simulink model "TST_ASMod_VolEff"  (R2016b)
settings: Solver=FixedStepDiscrete  StartTime=0.0  StopTime=simTime  FixedStep=sampleTime  RelTol=1e-3
values from neighbouring files (symbols this model uses):
  testCase = 1    [initTST_ASMod_VolEff_001.m]
libraries: simulink x5, UnitTest_Lib x3
settings Model: Creator=bianxuyin  LastModifiedBy=bianxuyin
settings DebuggingCC: SignalRangeChecking=error

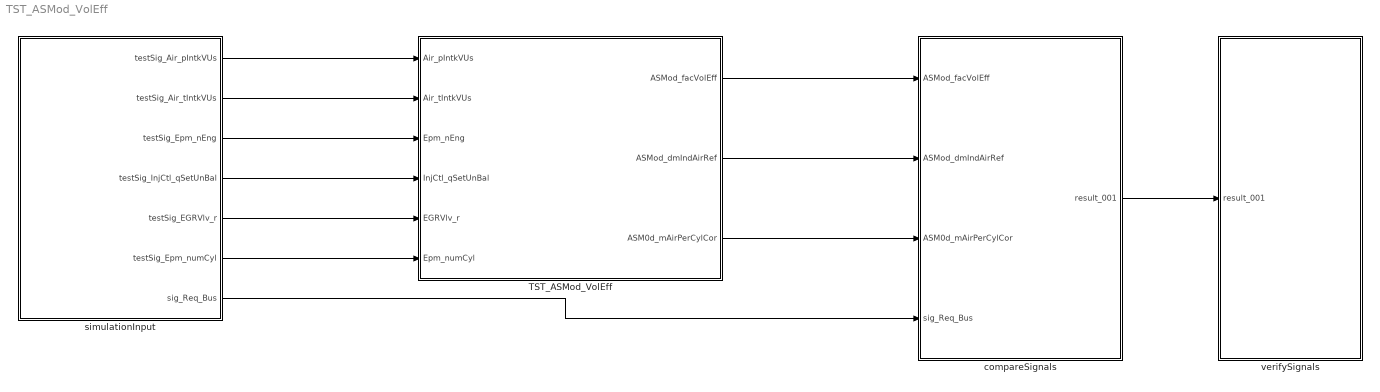
== system TST_ASMod_VolEff ==
  TST_ASMod_VolEff : Subsystem
  compareSignals : Subsystem
  simulationInput : Subsystem
  verifySignals : Subsystem
  wires:
  simulationInput/1(testSig_Air_pIntkVUs) -> TST_ASMod_VolEff/1(Air_pIntkVUs)
  simulationInput/2(testSig_Air_tIntkVUs) -> TST_ASMod_VolEff/2(Air_tIntkVUs)
  simulationInput/3(testSig_Epm_nEng) -> TST_ASMod_VolEff/3(Epm_nEng)
  simulationInput/4(testSig_InjCtl_qSetUnBal) -> TST_ASMod_VolEff/4(InjCtl_qSetUnBal)
  simulationInput/5(testSig_EGRVlv_r) -> TST_ASMod_VolEff/5(EGRVlv_r)
  simulationInput/6(testSig_Epm_numCyl) -> TST_ASMod_VolEff/6(Epm_numCyl)
  TST_ASMod_VolEff/1(ASMod_facVolEff) -> compareSignals/1(ASMod_facVolEff)
  TST_ASMod_VolEff/2(ASMod_dmIndAirRef) -> compareSignals/2(ASMod_dmIndAirRef)
  TST_ASMod_VolEff/3(ASM0d_mAirPerCylCor) -> compareSignals/3(ASM0d_mAirPerCylCor)
  simulationInput/7(sig_Req_Bus) -> compareSignals/4(sig_Req_Bus)
  compareSignals/1(result_001) -> verifySignals/1(result_001)

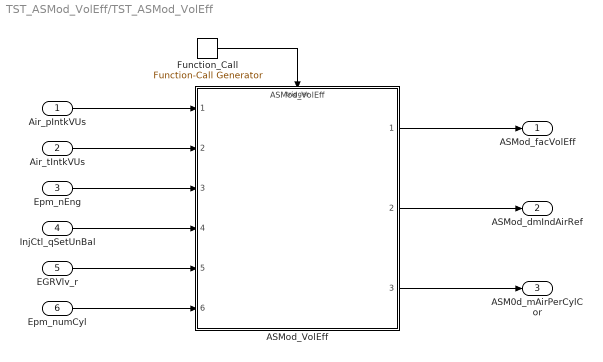
== system TST_ASMod_VolEff/TST_ASMod_VolEff ==
  Air_pIntkVUs : Inport
  Air_tIntkVUs : Inport  Port=2
  Epm_nEng : Inport  Port=3
  InjCtl_qSetUnBal : Inport  Port=4
  EGRVlv_r : Inport  Port=5
  Epm_numCyl : Inport  Port=6
  ASMod_VolEff : ModelReference  ModelNameDialog=ASMod_VolEff  SimulationMode=Normal  ModelReferenceVersion=1.20  TriggerPortName=function  TriggerPortTriggerType=function-call  TriggerPortStatesWhenEnabling=held
  Function_Call : simulink/Ports & Subsystems/Function-Call Generator  sample_time=sampleTime  numberOfIterations=1
  ASMod_facVolEff : Outport
  ASMod_dmIndAirRef : Outport  Port=2
  ASM0d_mAirPerCylCor : Outport  Port=3
  wires:
  Function_Call/1 -> ASMod_VolEff/Trigger
  Air_pIntkVUs/1 -> ASMod_VolEff/1
  Air_tIntkVUs/1 -> ASMod_VolEff/2
  Epm_nEng/1 -> ASMod_VolEff/3
  InjCtl_qSetUnBal/1 -> ASMod_VolEff/4
  EGRVlv_r/1 -> ASMod_VolEff/5
  Epm_numCyl/1 -> ASMod_VolEff/6
  ASMod_VolEff/1 -> ASMod_facVolEff/1
  ASMod_VolEff/2 -> ASMod_dmIndAirRef/1
  ASMod_VolEff/3 -> ASM0d_mAirPerCylCor/1

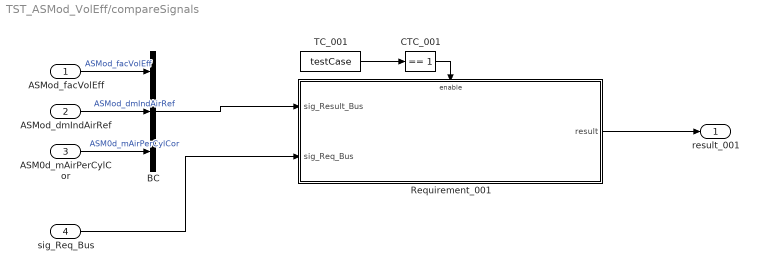
== system TST_ASMod_VolEff/compareSignals ==
  ASMod_facVolEff : Inport
  ASMod_dmIndAirRef : Inport  Port=2
  ASM0d_mAirPerCylCor : Inport  Port=3
  sig_Req_Bus : Inport  Port=4
  BC : BusCreator  Inputs=3
  CTC_001 : simulink/Logic and Bit Operations/Compare To Constant  relop===  const=1  OutDataTypeStr=boolean
  Requirement_001 : Subsystem
  TC_001 : Constant  Value=testCase
  result_001 : Outport
  wires:
  ASMod_facVolEff/1 -> BC/1  "ASMod_facVolEff"
  ASMod_dmIndAirRef/1 -> BC/2  "ASMod_dmIndAirRef"
  ASM0d_mAirPerCylCor/1 -> BC/3  "ASM0d_mAirPerCylCor"
  TC_001/1 -> CTC_001/1
  CTC_001/1 -> Requirement_001/Enable
  sig_Req_Bus/1 -> Requirement_001/2(sig_Req_Bus)
  BC/1 -> Requirement_001/1(sig_Result_Bus)
  Requirement_001/1(result) -> result_001/1

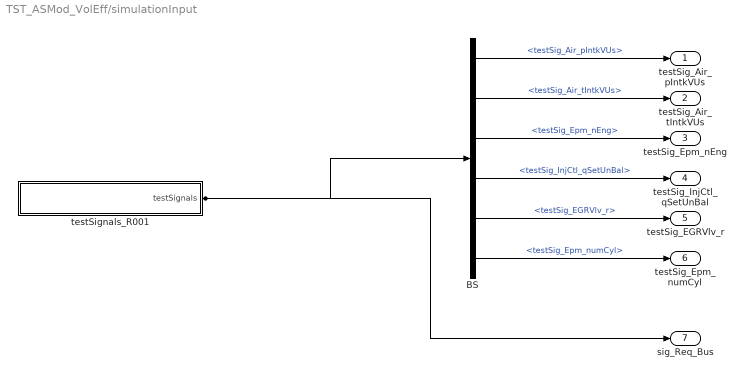
== system TST_ASMod_VolEff/simulationInput ==
  BS : BusSelector  OutputSignals=testSig_Air_pIntkVUs,testSig_Air_tIntkVUs,testSig_Epm_nEng,testSig_InjCtl_qSetUnBal,testSig_EGRVlv_r,testSig_Epm_numCyl
  testSignals_R001 : Subsystem
  testSig_Air_pIntkVUs : Outport
  testSig_Air_tIntkVUs : Outport  Port=2
  testSig_Epm_nEng : Outport  Port=3
  testSig_InjCtl_qSetUnBal : Outport  Port=4
  testSig_EGRVlv_r : Outport  Port=5
  testSig_Epm_numCyl : Outport  Port=6
  sig_Req_Bus : Outport  Port=7
  wires:
  BS/1 -> testSig_Air_pIntkVUs/1  "<testSig_Air_pIntkVUs>"
  BS/2 -> testSig_Air_tIntkVUs/1  "<testSig_Air_tIntkVUs>"
  BS/3 -> testSig_Epm_nEng/1  "<testSig_Epm_nEng>"
  BS/4 -> testSig_InjCtl_qSetUnBal/1  "<testSig_InjCtl_qSetUnBal>"
  BS/5 -> testSig_EGRVlv_r/1  "<testSig_EGRVlv_r>"
  BS/6 -> testSig_Epm_numCyl/1  "<testSig_Epm_numCyl>"
  testSignals_R001/1(testSignals) -> BS/1, sig_Req_Bus/1

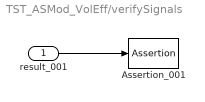
== system TST_ASMod_VolEff/verifySignals ==
  result_001 : Inport
  Assertion_001 : Assertion  Enabled=off
  wires:
  result_001/1 -> Assertion_001/1

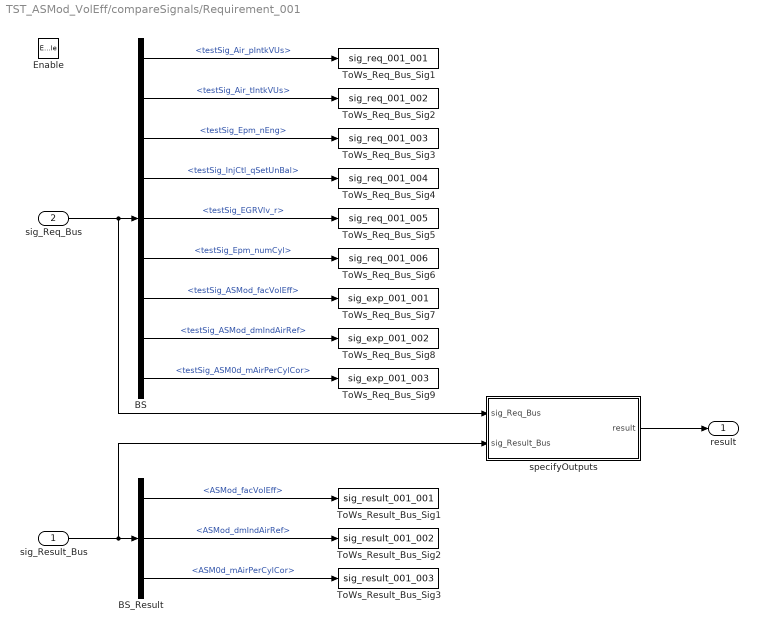
== system TST_ASMod_VolEff/compareSignals/Requirement_001 ==
  sig_Result_Bus : Inport
  sig_Req_Bus : Inport  Port=2
  Enable : EnablePort
  BS : BusSelector  OutputSignals=testSig_Air_pIntkVUs,testSig_Air_tIntkVUs,testSig_Epm_nEng,testSig_InjCtl_qSetUnBal,testSig_EGRVlv_r,testSig_Epm_numCyl,testSig_ASMod_facVolEff,testSig_ASMod_dmIndAirRef,testSig_ASM0d_mAirPerCylCor
  BS_Result : BusSelector  OutputSignals=ASMod_facVolEff,ASMod_dmIndAirRef,ASM0d_mAirPerCylCor
  ToWs_Req_Bus_Sig1 : ToWorkspace  VariableName=sig_req_001_001  SaveFormat=Structure With Time
  ToWs_Req_Bus_Sig2 : ToWorkspace  VariableName=sig_req_001_002  SaveFormat=Structure With Time
  ToWs_Req_Bus_Sig3 : ToWorkspace  VariableName=sig_req_001_003  SaveFormat=Structure With Time
  ToWs_Req_Bus_Sig4 : ToWorkspace  VariableName=sig_req_001_004  SaveFormat=Structure With Time
  ToWs_Req_Bus_Sig5 : ToWorkspace  VariableName=sig_req_001_005  SaveFormat=Structure With Time
  ToWs_Req_Bus_Sig6 : ToWorkspace  VariableName=sig_req_001_006  SaveFormat=Structure With Time
  ToWs_Req_Bus_Sig7 : ToWorkspace  VariableName=sig_exp_001_001  SaveFormat=Structure With Time
  ToWs_Req_Bus_Sig8 : ToWorkspace  VariableName=sig_exp_001_002  SaveFormat=Structure With Time
  ToWs_Req_Bus_Sig9 : ToWorkspace  VariableName=sig_exp_001_003  SaveFormat=Structure With Time
  ToWs_Result_Bus_Sig1 : ToWorkspace  VariableName=sig_result_001_001  SaveFormat=Structure With Time
  ToWs_Result_Bus_Sig2 : ToWorkspace  VariableName=sig_result_001_002  SaveFormat=Structure With Time
  ToWs_Result_Bus_Sig3 : ToWorkspace  VariableName=sig_result_001_003  SaveFormat=Structure With Time
  specifyOutputs : Subsystem
  result : Outport
  wires:
  sig_Req_Bus/1 -> BS/1, specifyOutputs/1(sig_Req_Bus)
  BS/1 -> ToWs_Req_Bus_Sig1/1  "<testSig_Air_pIntkVUs>"
  BS/2 -> ToWs_Req_Bus_Sig2/1  "<testSig_Air_tIntkVUs>"
  BS/3 -> ToWs_Req_Bus_Sig3/1  "<testSig_Epm_nEng>"
  BS/4 -> ToWs_Req_Bus_Sig4/1  "<testSig_InjCtl_qSetUnBal>"
  BS/5 -> ToWs_Req_Bus_Sig5/1  "<testSig_EGRVlv_r>"
  BS/6 -> ToWs_Req_Bus_Sig6/1  "<testSig_Epm_numCyl>"
  BS/7 -> ToWs_Req_Bus_Sig7/1  "<testSig_ASMod_facVolEff>"
  BS/8 -> ToWs_Req_Bus_Sig8/1  "<testSig_ASMod_dmIndAirRef>"
  BS/9 -> ToWs_Req_Bus_Sig9/1  "<testSig_ASM0d_mAirPerCylCor>"
  sig_Result_Bus/1 -> BS_Result/1, specifyOutputs/2(sig_Result_Bus)
  BS_Result/1 -> ToWs_Result_Bus_Sig1/1  "<ASMod_facVolEff>"
  BS_Result/2 -> ToWs_Result_Bus_Sig2/1  "<ASMod_dmIndAirRef>"
  BS_Result/3 -> ToWs_Result_Bus_Sig3/1  "<ASM0d_mAirPerCylCor>"
  specifyOutputs/1(result) -> result/1

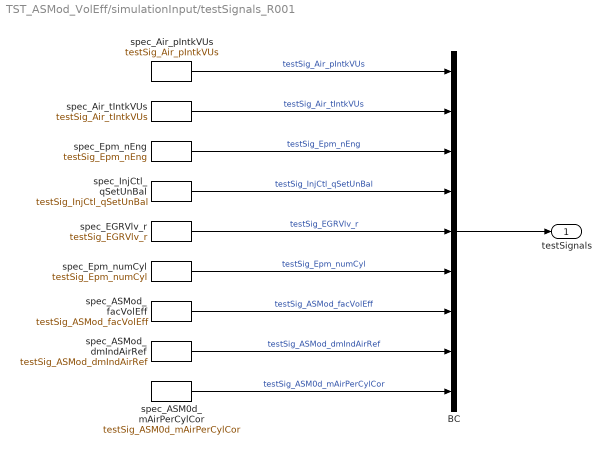
== system TST_ASMod_VolEff/simulationInput/testSignals_R001 ==
  BC : BusCreator  Inputs=9
  spec_ASM0d_mAirPerCylCor : FromWorkspace  VariableName=testSig_ASM0d_mAirPerCylCor  Interpolate=off  OutputAfterFinalValue=Holding final value
  spec_ASMod_dmIndAirRef : FromWorkspace  VariableName=testSig_ASMod_dmIndAirRef  Interpolate=off  OutputAfterFinalValue=Holding final value
  spec_ASMod_facVolEff : FromWorkspace  VariableName=testSig_ASMod_facVolEff  Interpolate=off  OutputAfterFinalValue=Holding final value
  spec_Air_pIntkVUs : FromWorkspace  VariableName=testSig_Air_pIntkVUs  Interpolate=off  OutputAfterFinalValue=Holding final value
  spec_Air_tIntkVUs : FromWorkspace  VariableName=testSig_Air_tIntkVUs  Interpolate=off  OutputAfterFinalValue=Holding final value
  spec_EGRVlv_r : FromWorkspace  VariableName=testSig_EGRVlv_r  Interpolate=off  OutputAfterFinalValue=Holding final value
  spec_Epm_nEng : FromWorkspace  VariableName=testSig_Epm_nEng  Interpolate=off  OutputAfterFinalValue=Holding final value
  spec_Epm_numCyl : FromWorkspace  VariableName=testSig_Epm_numCyl  Interpolate=off  OutputAfterFinalValue=Holding final value
  spec_InjCtl_qSetUnBal : FromWorkspace  VariableName=testSig_InjCtl_qSetUnBal  Interpolate=off  OutputAfterFinalValue=Holding final value
  testSignals : Outport
  wires:
  BC/1 -> testSignals/1
  spec_Air_pIntkVUs/1 -> BC/1  "testSig_Air_pIntkVUs"
  spec_Air_tIntkVUs/1 -> BC/2  "testSig_Air_tIntkVUs"
  spec_Epm_nEng/1 -> BC/3  "testSig_Epm_nEng"
  spec_InjCtl_qSetUnBal/1 -> BC/4  "testSig_InjCtl_qSetUnBal"
  spec_EGRVlv_r/1 -> BC/5  "testSig_EGRVlv_r"
  spec_Epm_numCyl/1 -> BC/6  "testSig_Epm_numCyl"
  spec_ASMod_facVolEff/1 -> BC/7  "testSig_ASMod_facVolEff"
  spec_ASMod_dmIndAirRef/1 -> BC/8  "testSig_ASMod_dmIndAirRef"
  spec_ASM0d_mAirPerCylCor/1 -> BC/9  "testSig_ASM0d_mAirPerCylCor"

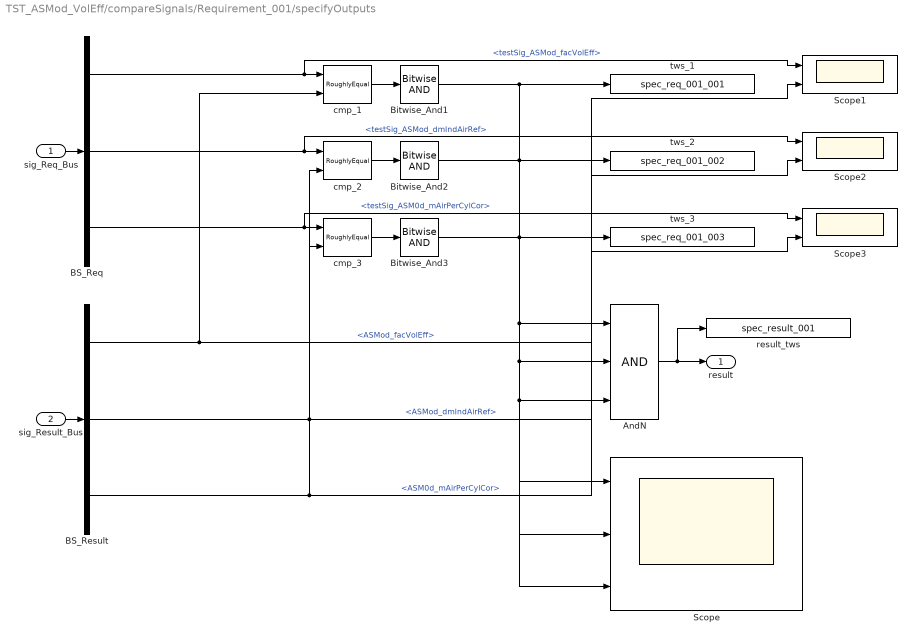
== system TST_ASMod_VolEff/compareSignals/Requirement_001/specifyOutputs ==
  sig_Req_Bus : Inport
  sig_Result_Bus : Inport  Port=2
  AndN : Logic  Inputs=3
  BS_Req : BusSelector  OutputSignals=testSig_ASMod_facVolEff,testSig_ASMod_dmIndAirRef,testSig_ASM0d_mAirPerCylCor
  BS_Result : BusSelector  OutputSignals=ASMod_facVolEff,ASMod_dmIndAirRef,ASM0d_mAirPerCylCor
  Bitwise_And1 : simulink/Logic and Bit Operations/Bitwise Operator  logicop=AND  UseBitMask=off  BitMask=bin2dec('11011001')  BitMaskRealWorld=Stored Integer
  Bitwise_And2 : simulink/Logic and Bit Operations/Bitwise Operator  logicop=AND  UseBitMask=off  BitMask=bin2dec('11011001')  BitMaskRealWorld=Stored Integer
  Bitwise_And3 : simulink/Logic and Bit Operations/Bitwise Operator  logicop=AND  UseBitMask=off  BitMask=bin2dec('11011001')  BitMaskRealWorld=Stored Integer
  Scope : Scope  NumInputPorts=3
  Scope1 : Scope  NumInputPorts=2
  Scope2 : Scope  NumInputPorts=2
  Scope3 : Scope  NumInputPorts=2
  cmp_1 : UnitTest_Lib/RoughlyEqual  slope=0.1
  cmp_2 : UnitTest_Lib/RoughlyEqual  slope=1
  cmp_3 : UnitTest_Lib/RoughlyEqual  slope=1
  result_tws : ToWorkspace  VariableName=spec_result_001
  tws_1 : ToWorkspace  VariableName=spec_req_001_001
  tws_2 : ToWorkspace  VariableName=spec_req_001_002
  tws_3 : ToWorkspace  VariableName=spec_req_001_003
  result : Outport
  wires:
  sig_Req_Bus/1 -> BS_Req/1
  sig_Result_Bus/1 -> BS_Result/1
  AndN/1 -> result/1, result_tws/1
  BS_Req/1 -> cmp_1/1, Scope1/1  "<testSig_ASMod_facVolEff>"
  BS_Result/1 -> cmp_1/2, Scope1/2  "<ASMod_facVolEff>"
  cmp_1/1 -> Bitwise_And1/1
  Bitwise_And1/1 -> AndN/1, Scope/1, tws_1/1
  BS_Req/2 -> cmp_2/1, Scope2/1  "<testSig_ASMod_dmIndAirRef>"
  BS_Result/2 -> cmp_2/2, Scope2/2  "<ASMod_dmIndAirRef>"
  cmp_2/1 -> Bitwise_And2/1
  Bitwise_And2/1 -> AndN/2, Scope/2, tws_2/1
  BS_Req/3 -> cmp_3/1, Scope3/1  "<testSig_ASM0d_mAirPerCylCor>"
  BS_Result/3 -> cmp_3/2, Scope3/2  "<ASM0d_mAirPerCylCor>"
  cmp_3/1 -> Bitwise_And3/1
  Bitwise_And3/1 -> AndN/3, Scope/3, tws_3/1
